simulink model "LQR_s_inv"  (R2023b)
settings: Solver=VariableStepAuto  StartTime=0.0  StopTime=10.0  RelTol=1e-3
values from neighbouring files (symbols this model uses):
  K = [k1 k2 ki]    [WP2.m]
settings Model: Creator=giova  LastModifiedBy=Principale

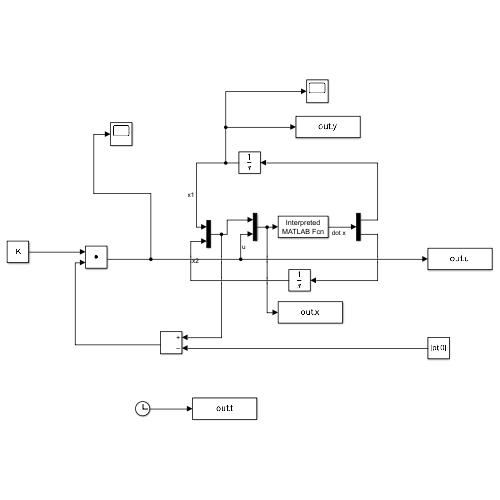
[thumbnail: Simulink's stored preview of the top-level diagram]
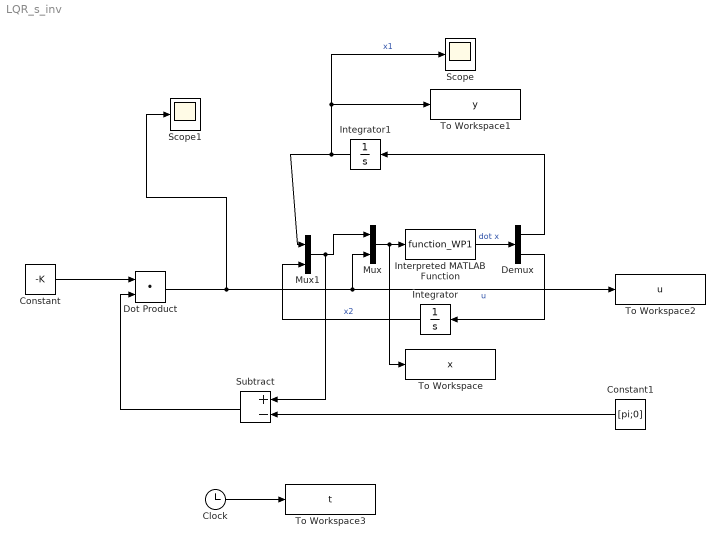
== system LQR_s_inv ==
  Clock : Clock
  Constant : Constant  Value=-K
  Constant1 : Constant  Value=[pi;0]
  Demux : Demux  Outputs=2
  Dot Product : DotProduct  OutDataTypeStr=Inherit: Inherit via internal rule
  Integrator : Integrator
  Integrator1 : Integrator
  Interpreted MATLAB Function : MATLABFcn  MATLABFcn=function_WP1  OutputDimensions=2
  Mux : Mux  Inputs=2
  Mux1 : Mux  Inputs=2
  Scope : Scope
  Scope1 : Scope
  Subtract : Sum  Inputs=+-
  To Workspace : ToWorkspace  VariableName=x  SampleTime=-1
  To Workspace1 : ToWorkspace  VariableName=y  SampleTime=-1
  To Workspace2 : ToWorkspace  VariableName=u  SampleTime=-1
  To Workspace3 : ToWorkspace  VariableName=t  SampleTime=-1
  wires:
  Integrator1/1 -> Scope/1, To Workspace1/1, Mux1/1  "x1"
  Mux/1 -> To Workspace/1, Interpreted MATLAB Function/1
  Interpreted MATLAB Function/1 -> Demux/1  "dot x"
  Mux1/1 -> Subtract/1, Mux/1
  Demux/1 -> Integrator1/1
  Integrator/1 -> Mux1/2  "x2"
  Demux/2 -> Integrator/1
  Constant/1 -> Dot Product/1
  Constant1/1 -> Subtract/2
  Subtract/1 -> Dot Product/2
  Dot Product/1 -> Scope1/1, Mux/2, To Workspace2/1  "u"
  Clock/1 -> To Workspace3/1
